simulink model "ACC_speed_change_curve_cs"  (R2016a)
settings: Solver=ode5  SolverMode=SingleTasking  StartTime=0.0  StopTime=inf  FixedStep=1/1000  RelTol=1e-3
PreLoadFcn:
  | mbxruntime.callbacks.PreLoadFcn(bdroot);
  | check_NUTS_defined;
  | 
  | assignin('base',['model_closed_' bdroot],false);addpath('../includes_ACC');
PostLoadFcn:
  | mbxruntime.callbacks.PostLoadFcn(bdroot);
InitFcn:
  | mbxruntime.callbacks.InitFcn(bdroot);
StartFcn:
  | mbxruntime.callbacks.StartFcn(bdroot);
StopFcn:
  | mbxruntime.callbacks.StopFcn(bdroot);
model workspace (MAT data in the model file):
  mbox_table : struct (value not decoded)
  model_closed = 0
  sim_status = 0
undefined symbols (not defined in the file or in its folder): DiscIntNeverNeededParam
undefined symbols (not defined in the file): SteeringColumn, SteeringWheel, WheelL0, WheelL1, WheelR0, WheelR1
libraries: simulink_extras x49, simulink x29, PreScanSimulinkLibrary x24, PreScanUsefulBlocks x2, Solver_SF x1, simulink_need_slupdate x1
(part 9 of 17)

== system ACC_speed_change_curve_cs/Toyota_Yaris_1/SteeringColumn_pivot_Mux ==
  X [m] : Inport
  Y [m] : Inport  Port=2
  Z [m] : Inport  Port=3
  Roll [rad] : Inport  Port=4
  Pitch [rad] : Inport  Port=5
  Yaw [rad] : Inport  Port=6
  Bus Creator : BusCreator  Inputs=3  OutDataTypeStr=Bus: PRESCAN_XYZ_DATA
  Bus Creator1 : BusCreator  Inputs=3  OutDataTypeStr=Bus: PRESCAN_RPY_DATA
  Bus Creator2 : BusCreator  Inputs=2  OutDataTypeStr=Bus: PRESCAN_POSE_DATA
  Joint : Outport
  wires:
  Yaw [rad]/1 -> Bus Creator1/3  "Yaw"
  Bus Creator1/1 -> Bus Creator2/2  "ORIENTATION"
  Bus Creator/1 -> Bus Creator2/1  "POSITION"
  X [m]/1 -> Bus Creator/1  "X"
  Y [m]/1 -> Bus Creator/2  "Y"
  Z [m]/1 -> Bus Creator/3  "Z"
  Bus Creator2/1 -> Joint/1
  Roll [rad]/1 -> Bus Creator1/1  "Roll"
  Pitch [rad]/1 -> Bus Creator1/2  "Pitch"

== system ACC_speed_change_curve_cs/Toyota_Yaris_1/SteeringWheel_pivot_Mux ==
  X [m] : Inport
  Y [m] : Inport  Port=2
  Z [m] : Inport  Port=3
  Roll [rad] : Inport  Port=4
  Pitch [rad] : Inport  Port=5
  Yaw [rad] : Inport  Port=6
  Bus Creator : BusCreator  Inputs=3  OutDataTypeStr=Bus: PRESCAN_XYZ_DATA
  Bus Creator1 : BusCreator  Inputs=3  OutDataTypeStr=Bus: PRESCAN_RPY_DATA
  Bus Creator2 : BusCreator  Inputs=2  OutDataTypeStr=Bus: PRESCAN_POSE_DATA
  Joint : Outport
  wires:
  Yaw [rad]/1 -> Bus Creator1/3  "Yaw"
  Bus Creator1/1 -> Bus Creator2/2  "ORIENTATION"
  Bus Creator/1 -> Bus Creator2/1  "POSITION"
  X [m]/1 -> Bus Creator/1  "X"
  Y [m]/1 -> Bus Creator/2  "Y"
  Z [m]/1 -> Bus Creator/3  "Z"
  Bus Creator2/1 -> Joint/1
  Roll [rad]/1 -> Bus Creator1/1  "Roll"
  Pitch [rad]/1 -> Bus Creator1/2  "Pitch"

== system ACC_speed_change_curve_cs/Toyota_Yaris_1/Trajectories ==
  Traj2State1 : Subsystem  Tag=Traj2State  mask(PreScan Demux Block:){}
      settings: DeleteFcn=PreScanBlockDeleteFcn;
  TrajCoGOffset : Subsystem  Tag=TrajCoGOffset  mask(Trajectory CoG Offset block){CoGOffsetZ=0.57, InitRoll=0, InitPitch=0}
      mask prompts: CoGOffsetZ "Z-component of CoG Offset [m]:"; InitRoll "Initial Roll angle [deg]:"; InitPitch "Initial Pitch angle [deg]:"
      mask help: A trajectory follows the surface of the road. However the position of a actor is based on the actor's Center of Gravity, which is typically above the road. This block converts from the trajectory along the road surface to the trajectory of the actor's CoG by realigning the z-component of the CoG offset to be normal to the road.
      settings: DeleteFcn=PreScanBlockDeleteFcn;
  Trajectory_4 : Subsystem  Tag=Trajectory  mask(PreScan Source Block: Trajectory){FileName='Trajectory_4.mat', TimeStep=20/1000}
      mask prompts: TimeStep "Time Step [s]"
      mask help:
      | The Trajectory block contains the trajectories defined in the PreScan Experiment Editor. The output of the trajectory block is the (vehicle) State.
      |
      | For more information, please click Help.
      mask init: same as ACC_speed_change_curve_cs/Audi_A8_1/Trajectories/Trajectory_1
      settings: DeleteFcn=PreScanBlockDeleteFcn;
      mask Help: eval('openHelp(312)')
      mask Display: fprintf(FileName)
  Trajectory_4_Offset : Constant  Tag=TrajectoryOffset  Value="[0  0  0  0  0  0]"
  State : Outport  Tag=TrajOutport
  wires:
  Trajectory_4/1(trajectory) -> Traj2State1/1(Traj Org)
  Trajectory_4_Offset/1 -> Traj2State1/2(Offset)
  TrajCoGOffset/1(State Out) -> State/1
  Traj2State1/1(state) -> TrajCoGOffset/1(State In)

== system ACC_speed_change_curve_cs/Toyota_Yaris_1/WheelDisplacement_Mux ==
  Steering Angle Front [rad] : Inport  Tag=inport/JointGroup  SampleTime=20/1000  BusOutputAsStruct=on
  Steering Angle Rear [rad] : Inport  Tag=inport/JointGroup  Port=2  SampleTime=20/1000  BusOutputAsStruct=on
  Rotation [rad] : Inport  Tag=inport/JointGroup  Port=3  SampleTime=20/1000  BusOutputAsStruct=on
  zDisp FL [m] : Inport  Tag=inport/JointGroup  Port=4  SampleTime=20/1000  BusOutputAsStruct=on
  zDisp FR [m] : Inport  Tag=inport/JointGroup  Port=5  SampleTime=20/1000  BusOutputAsStruct=on
  zDisp RL [m] : Inport  Tag=inport/JointGroup  Port=6  SampleTime=20/1000  BusOutputAsStruct=on
  zDisp RR [m] : Inport  Tag=inport/JointGroup  Port=7  SampleTime=20/1000  BusOutputAsStruct=on
  Ground_{1..12} (12 alike) : Ground
  WheelL0_Mux : Subsystem  Tag=mux/Joint  mask(PreScan Mux Block){DisplayName=WheelL0}
      mask prompts: DisplayName "Display Name"
      mask help:
      | This block simulates a generic joint used for generic models. This joint can be enabled/disabled from the GUI.
      |
      | For more information, please click Help.
      settings: DeleteFcn=PreScanBlockDeleteFcn;
      mask Help: eval('openHelp(254)')
  WheelL1_Mux : Subsystem  Tag=mux/Joint  mask(PreScan Mux Block){DisplayName=WheelL1}
      mask prompts: DisplayName "Display Name"
      mask help:
      | This block simulates a generic joint used for generic models. This joint can be enabled/disabled from the GUI.
      |
      | For more information, please click Help.
      settings: DeleteFcn=PreScanBlockDeleteFcn;
      mask Help: eval('openHelp(254)')
  WheelR0_Mux : Subsystem  Tag=mux/Joint  mask(PreScan Mux Block){DisplayName=WheelR0}
      mask prompts: DisplayName "Display Name"
      mask help:
      | This block simulates a generic joint used for generic models. This joint can be enabled/disabled from the GUI.
      |
      | For more information, please click Help.
      settings: DeleteFcn=PreScanBlockDeleteFcn;
      mask Help: eval('openHelp(254)')
  WheelR1_Mux : Subsystem  Tag=mux/Joint  mask(PreScan Mux Block){DisplayName=WheelR1}
      mask prompts: DisplayName "Display Name"
      mask help:
      | This block simulates a generic joint used for generic models. This joint can be enabled/disabled from the GUI.
      |
      | For more information, please click Help.
      settings: DeleteFcn=PreScanBlockDeleteFcn;
      mask Help: eval('openHelp(254)')
  WheelL0_Toyota_Yaris_1 : Outport  Tag=outport/JointActuator  OutDataTypeStr=Bus: PRESCAN_POSE_DATA  SampleTime=20/1000
  WheelL1_Toyota_Yaris_1 : Outport  Tag=outport/JointActuator  Port=2  OutDataTypeStr=Bus: PRESCAN_POSE_DATA  SampleTime=20/1000
  WheelR0_Toyota_Yaris_1 : Outport  Tag=outport/JointActuator  Port=3  OutDataTypeStr=Bus: PRESCAN_POSE_DATA  SampleTime=20/1000
  WheelR1_Toyota_Yaris_1 : Outport  Tag=outport/JointActuator  Port=4  OutDataTypeStr=Bus: PRESCAN_POSE_DATA  SampleTime=20/1000
  wires:
  WheelL0_Mux/1(Joint) -> WheelL0_Toyota_Yaris_1/1
  WheelL1_Mux/1(Joint) -> WheelL1_Toyota_Yaris_1/1
  WheelR0_Mux/1(Joint) -> WheelR0_Toyota_Yaris_1/1
  WheelR1_Mux/1(Joint) -> WheelR1_Toyota_Yaris_1/1
  Steering Angle Front [rad]/1 -> WheelR0_Mux/6(Yaw [rad]), WheelL0_Mux/6(Yaw [rad])
  Steering Angle Rear [rad]/1 -> WheelR1_Mux/6(Yaw [rad]), WheelL1_Mux/6(Yaw [rad])
  Rotation [rad]/1 -> WheelR0_Mux/5(Pitch [rad]), WheelL0_Mux/5(Pitch [rad]), WheelR1_Mux/5(Pitch [rad]), WheelL1_Mux/5(Pitch [rad])
  zDisp FL [m]/1 -> WheelL0_Mux/3(Z [m])
  zDisp FR [m]/1 -> WheelR0_Mux/3(Z [m])
  zDisp RL [m]/1 -> WheelL1_Mux/3(Z [m])
  zDisp RR [m]/1 -> WheelR1_Mux/3(Z [m])
  Ground_1/1 -> WheelL0_Mux/1(X [m])
  Ground_2/1 -> WheelL0_Mux/2(Y [m])
  Ground_3/1 -> WheelL0_Mux/4(Roll [rad])
  Ground_4/1 -> WheelL1_Mux/1(X [m])
  Ground_5/1 -> WheelL1_Mux/2(Y [m])
  Ground_6/1 -> WheelL1_Mux/4(Roll [rad])
  Ground_7/1 -> WheelR0_Mux/1(X [m])
  Ground_8/1 -> WheelR0_Mux/2(Y [m])
  Ground_9/1 -> WheelR0_Mux/4(Roll [rad])
  Ground_10/1 -> WheelR1_Mux/1(X [m])
  Ground_11/1 -> WheelR1_Mux/2(Y [m])
  Ground_12/1 -> WheelR1_Mux/4(Roll [rad])

== system ACC_speed_change_curve_cs/Toyota_Yaris_1/d2r SteeringColumn_pivot_Mux ==
  Degrees in : Inport
  Gain1 : Gain  Gain=pi/180  SaturateOnIntegerOverflow=on  OutDataTypeStr=Inherit: Same as input  ParamDataTypeStr=Inherit: Same as input
  Radians out : Outport  InitialOutput=0
  wires:
  Gain1/1 -> Radians out/1
  Degrees in/1 -> Gain1/1

== system ACC_speed_change_curve_cs/Toyota_Yaris_1/d2r SteeringWheel_pivot_Mux ==
  Degrees in : Inport
  Gain1 : Gain  Gain=pi/180  SaturateOnIntegerOverflow=on  OutDataTypeStr=Inherit: Same as input  ParamDataTypeStr=Inherit: Same as input
  Radians out : Outport  InitialOutput=0
  wires:
  Gain1/1 -> Radians out/1
  Degrees in/1 -> Gain1/1

== system ACC_speed_change_curve_cs/Toyota_Yaris_1/d2r WheelDisplacement_Mux 1 ==
  Degrees in : Inport
  Gain1 : Gain  Gain=pi/180  SaturateOnIntegerOverflow=on  OutDataTypeStr=Inherit: Same as input  ParamDataTypeStr=Inherit: Same as input
  Radians out : Outport  InitialOutput=0
  wires:
  Gain1/1 -> Radians out/1
  Degrees in/1 -> Gain1/1

== system ACC_speed_change_curve_cs/Toyota_Yaris_1/d2r WheelDisplacement_Mux 2 ==
  Degrees in : Inport
  Gain1 : Gain  Gain=pi/180  SaturateOnIntegerOverflow=on  OutDataTypeStr=Inherit: Same as input  ParamDataTypeStr=Inherit: Same as input
  Radians out : Outport  InitialOutput=0
  wires:
  Gain1/1 -> Radians out/1
  Degrees in/1 -> Gain1/1

== system ACC_speed_change_curve_cs/WheelL0_Audi_A8_1/Actuator ==
  Joint : Inport
  Bus Selector : BusSelector  OutputSignals=POSITION,ORIENTATION
  visu_Rotate : Subsystem  mask(RPYActuator){UniqueID=UniqueID, Object3DID=Rotate_ObjectID3D, TimeStep=TimeStep}
      mask prompts: UniqueID "Auto-Assigned: Unique ID"; Object3DID "Auto-Assigned: Child 3D Object ID"; TimeStep "Auto-Assigned: Upload Period [s]"
      mask help: Applies angles update to selected child object
      mask Help:
      | Applies position update to selected child object
      | 
      | - UniqueID (double)   : Unique ID of the parent actor
      | - Object3DID (string) : Name of the child 3D object
      mask Display: port_label('input', 1, ['visu_Rotate_' Object3DID])
  visu_Translate : Subsystem  mask(PositionActuator){UniqueID=UniqueID, Object3DID=Translate_ObjectID3D, TimeStep=TimeStep}
      mask prompts: UniqueID "Auto-Assigned: Unique ID"; Object3DID "Auto-Assigned: Child 3D Object ID"; TimeStep "Auto-Assigned: Upload Period [s]"
      mask help: Applies position update to selected child object
      mask Help:
      | Applies position update to selected child object
      | 
      | - UniqueID (double)   : Unique ID of the parent actor
      | - Object3DID (string) : Name of the child 3D object
      mask Display: port_label('input', 1, ['visu_Translate_' Object3DID])
  wires:
  Bus Selector/2 -> visu_Rotate/1(In1)  "<ORIENTATION>"
  Bus Selector/1 -> visu_Translate/1(In1)  "<POSITION>"
  Joint/1 -> Bus Selector/1

== system ACC_speed_change_curve_cs/WheelL0_BMW_X5_1/Actuator ==
  Joint : Inport
  Bus Selector : BusSelector  OutputSignals=POSITION,ORIENTATION
  visu_Rotate : Subsystem  mask(RPYActuator){UniqueID=UniqueID, Object3DID=Rotate_ObjectID3D, TimeStep=TimeStep}
      mask prompts: UniqueID "Auto-Assigned: Unique ID"; Object3DID "Auto-Assigned: Child 3D Object ID"; TimeStep "Auto-Assigned: Upload Period [s]"
      mask help: Applies angles update to selected child object
      mask Help:
      | Applies position update to selected child object
      | 
      | - UniqueID (double)   : Unique ID of the parent actor
      | - Object3DID (string) : Name of the child 3D object
      mask Display: port_label('input', 1, ['visu_Rotate_' Object3DID])
  visu_Translate : Subsystem  mask(PositionActuator){UniqueID=UniqueID, Object3DID=Translate_ObjectID3D, TimeStep=TimeStep}
      mask prompts: UniqueID "Auto-Assigned: Unique ID"; Object3DID "Auto-Assigned: Child 3D Object ID"; TimeStep "Auto-Assigned: Upload Period [s]"
      mask help: Applies position update to selected child object
      mask Help:
      | Applies position update to selected child object
      | 
      | - UniqueID (double)   : Unique ID of the parent actor
      | - Object3DID (string) : Name of the child 3D object
      mask Display: port_label('input', 1, ['visu_Translate_' Object3DID])
  wires:
  Bus Selector/2 -> visu_Rotate/1(In1)  "<ORIENTATION>"
  Bus Selector/1 -> visu_Translate/1(In1)  "<POSITION>"
  Joint/1 -> Bus Selector/1

== system ACC_speed_change_curve_cs/WheelL0_Toyota_Previa_1/Actuator ==
  Joint : Inport
  Bus Selector : BusSelector  OutputSignals=POSITION,ORIENTATION
  visu_Rotate : Subsystem  mask(RPYActuator){UniqueID=UniqueID, Object3DID=Rotate_ObjectID3D, TimeStep=TimeStep}
      mask prompts: UniqueID "Auto-Assigned: Unique ID"; Object3DID "Auto-Assigned: Child 3D Object ID"; TimeStep "Auto-Assigned: Upload Period [s]"
      mask help: Applies angles update to selected child object
      mask Help:
      | Applies position update to selected child object
      | 
      | - UniqueID (double)   : Unique ID of the parent actor
      | - Object3DID (string) : Name of the child 3D object
      mask Display: port_label('input', 1, ['visu_Rotate_' Object3DID])
  visu_Translate : Subsystem  mask(PositionActuator){UniqueID=UniqueID, Object3DID=Translate_ObjectID3D, TimeStep=TimeStep}
      mask prompts: UniqueID "Auto-Assigned: Unique ID"; Object3DID "Auto-Assigned: Child 3D Object ID"; TimeStep "Auto-Assigned: Upload Period [s]"
      mask help: Applies position update to selected child object
      mask Help:
      | Applies position update to selected child object
      | 
      | - UniqueID (double)   : Unique ID of the parent actor
      | - Object3DID (string) : Name of the child 3D object
      mask Display: port_label('input', 1, ['visu_Translate_' Object3DID])
  wires:
  Bus Selector/2 -> visu_Rotate/1(In1)  "<ORIENTATION>"
  Bus Selector/1 -> visu_Translate/1(In1)  "<POSITION>"
  Joint/1 -> Bus Selector/1

== system ACC_speed_change_curve_cs/WheelL0_Toyota_Yaris_1/Actuator ==
  Joint : Inport
  Bus Selector : BusSelector  OutputSignals=POSITION,ORIENTATION
  visu_Rotate : Subsystem  mask(RPYActuator){UniqueID=UniqueID, Object3DID=Rotate_ObjectID3D, TimeStep=TimeStep}
      mask prompts: UniqueID "Auto-Assigned: Unique ID"; Object3DID "Auto-Assigned: Child 3D Object ID"; TimeStep "Auto-Assigned: Upload Period [s]"
      mask help: Applies angles update to selected child object
      mask Help:
      | Applies position update to selected child object
      | 
      | - UniqueID (double)   : Unique ID of the parent actor
      | - Object3DID (string) : Name of the child 3D object
      mask Display: port_label('input', 1, ['visu_Rotate_' Object3DID])
  visu_Translate : Subsystem  mask(PositionActuator){UniqueID=UniqueID, Object3DID=Translate_ObjectID3D, TimeStep=TimeStep}
      mask prompts: UniqueID "Auto-Assigned: Unique ID"; Object3DID "Auto-Assigned: Child 3D Object ID"; TimeStep "Auto-Assigned: Upload Period [s]"
      mask help: Applies position update to selected child object
      mask Help:
      | Applies position update to selected child object
      | 
      | - UniqueID (double)   : Unique ID of the parent actor
      | - Object3DID (string) : Name of the child 3D object
      mask Display: port_label('input', 1, ['visu_Translate_' Object3DID])
  wires:
  Bus Selector/2 -> visu_Rotate/1(In1)  "<ORIENTATION>"
  Bus Selector/1 -> visu_Translate/1(In1)  "<POSITION>"
  Joint/1 -> Bus Selector/1

== system ACC_speed_change_curve_cs/WheelL1_Audi_A8_1/Actuator ==
  Joint : Inport
  Bus Selector : BusSelector  OutputSignals=POSITION,ORIENTATION
  visu_Rotate : Subsystem  mask(RPYActuator){UniqueID=UniqueID, Object3DID=Rotate_ObjectID3D, TimeStep=TimeStep}
      mask prompts: UniqueID "Auto-Assigned: Unique ID"; Object3DID "Auto-Assigned: Child 3D Object ID"; TimeStep "Auto-Assigned: Upload Period [s]"
      mask help: Applies angles update to selected child object
      mask Help:
      | Applies position update to selected child object
      | 
      | - UniqueID (double)   : Unique ID of the parent actor
      | - Object3DID (string) : Name of the child 3D object
      mask Display: port_label('input', 1, ['visu_Rotate_' Object3DID])
  visu_Translate : Subsystem  mask(PositionActuator){UniqueID=UniqueID, Object3DID=Translate_ObjectID3D, TimeStep=TimeStep}
      mask prompts: UniqueID "Auto-Assigned: Unique ID"; Object3DID "Auto-Assigned: Child 3D Object ID"; TimeStep "Auto-Assigned: Upload Period [s]"
      mask help: Applies position update to selected child object
      mask Help:
      | Applies position update to selected child object
      | 
      | - UniqueID (double)   : Unique ID of the parent actor
      | - Object3DID (string) : Name of the child 3D object
      mask Display: port_label('input', 1, ['visu_Translate_' Object3DID])
  wires:
  Bus Selector/2 -> visu_Rotate/1(In1)  "<ORIENTATION>"
  Bus Selector/1 -> visu_Translate/1(In1)  "<POSITION>"
  Joint/1 -> Bus Selector/1

== system ACC_speed_change_curve_cs/WheelL1_BMW_X5_1/Actuator ==
  Joint : Inport
  Bus Selector : BusSelector  OutputSignals=POSITION,ORIENTATION
  visu_Rotate : Subsystem  mask(RPYActuator){UniqueID=UniqueID, Object3DID=Rotate_ObjectID3D, TimeStep=TimeStep}
      mask prompts: UniqueID "Auto-Assigned: Unique ID"; Object3DID "Auto-Assigned: Child 3D Object ID"; TimeStep "Auto-Assigned: Upload Period [s]"
      mask help: Applies angles update to selected child object
      mask Help:
      | Applies position update to selected child object
      | 
      | - UniqueID (double)   : Unique ID of the parent actor
      | - Object3DID (string) : Name of the child 3D object
      mask Display: port_label('input', 1, ['visu_Rotate_' Object3DID])
  visu_Translate : Subsystem  mask(PositionActuator){UniqueID=UniqueID, Object3DID=Translate_ObjectID3D, TimeStep=TimeStep}
      mask prompts: UniqueID "Auto-Assigned: Unique ID"; Object3DID "Auto-Assigned: Child 3D Object ID"; TimeStep "Auto-Assigned: Upload Period [s]"
      mask help: Applies position update to selected child object
      mask Help:
      | Applies position update to selected child object
      | 
      | - UniqueID (double)   : Unique ID of the parent actor
      | - Object3DID (string) : Name of the child 3D object
      mask Display: port_label('input', 1, ['visu_Translate_' Object3DID])
  wires:
  Bus Selector/2 -> visu_Rotate/1(In1)  "<ORIENTATION>"
  Bus Selector/1 -> visu_Translate/1(In1)  "<POSITION>"
  Joint/1 -> Bus Selector/1

== system ACC_speed_change_curve_cs/WheelL1_Toyota_Previa_1/Actuator ==
  Joint : Inport
  Bus Selector : BusSelector  OutputSignals=POSITION,ORIENTATION
  visu_Rotate : Subsystem  mask(RPYActuator){UniqueID=UniqueID, Object3DID=Rotate_ObjectID3D, TimeStep=TimeStep}
      mask prompts: UniqueID "Auto-Assigned: Unique ID"; Object3DID "Auto-Assigned: Child 3D Object ID"; TimeStep "Auto-Assigned: Upload Period [s]"
      mask help: Applies angles update to selected child object
      mask Help:
      | Applies position update to selected child object
      | 
      | - UniqueID (double)   : Unique ID of the parent actor
      | - Object3DID (string) : Name of the child 3D object
      mask Display: port_label('input', 1, ['visu_Rotate_' Object3DID])
  visu_Translate : Subsystem  mask(PositionActuator){UniqueID=UniqueID, Object3DID=Translate_ObjectID3D, TimeStep=TimeStep}
      mask prompts: UniqueID "Auto-Assigned: Unique ID"; Object3DID "Auto-Assigned: Child 3D Object ID"; TimeStep "Auto-Assigned: Upload Period [s]"
      mask help: Applies position update to selected child object
      mask Help:
      | Applies position update to selected child object
      | 
      | - UniqueID (double)   : Unique ID of the parent actor
      | - Object3DID (string) : Name of the child 3D object
      mask Display: port_label('input', 1, ['visu_Translate_' Object3DID])
  wires:
  Bus Selector/2 -> visu_Rotate/1(In1)  "<ORIENTATION>"
  Bus Selector/1 -> visu_Translate/1(In1)  "<POSITION>"
  Joint/1 -> Bus Selector/1

== system ACC_speed_change_curve_cs/WheelL1_Toyota_Yaris_1/Actuator ==
  Joint : Inport
  Bus Selector : BusSelector  OutputSignals=POSITION,ORIENTATION
  visu_Rotate : Subsystem  mask(RPYActuator){UniqueID=UniqueID, Object3DID=Rotate_ObjectID3D, TimeStep=TimeStep}
      mask prompts: UniqueID "Auto-Assigned: Unique ID"; Object3DID "Auto-Assigned: Child 3D Object ID"; TimeStep "Auto-Assigned: Upload Period [s]"
      mask help: Applies angles update to selected child object
      mask Help:
      | Applies position update to selected child object
      | 
      | - UniqueID (double)   : Unique ID of the parent actor
      | - Object3DID (string) : Name of the child 3D object
      mask Display: port_label('input', 1, ['visu_Rotate_' Object3DID])
  visu_Translate : Subsystem  mask(PositionActuator){UniqueID=UniqueID, Object3DID=Translate_ObjectID3D, TimeStep=TimeStep}
      mask prompts: UniqueID "Auto-Assigned: Unique ID"; Object3DID "Auto-Assigned: Child 3D Object ID"; TimeStep "Auto-Assigned: Upload Period [s]"
      mask help: Applies position update to selected child object
      mask Help:
      | Applies position update to selected child object
      | 
      | - UniqueID (double)   : Unique ID of the parent actor
      | - Object3DID (string) : Name of the child 3D object
      mask Display: port_label('input', 1, ['visu_Translate_' Object3DID])
  wires:
  Bus Selector/2 -> visu_Rotate/1(In1)  "<ORIENTATION>"
  Bus Selector/1 -> visu_Translate/1(In1)  "<POSITION>"
  Joint/1 -> Bus Selector/1

== system ACC_speed_change_curve_cs/WheelR0_Audi_A8_1/Actuator ==
  Joint : Inport
  Bus Selector : BusSelector  OutputSignals=POSITION,ORIENTATION
  visu_Rotate : Subsystem  mask(RPYActuator){UniqueID=UniqueID, Object3DID=Rotate_ObjectID3D, TimeStep=TimeStep}
      mask prompts: UniqueID "Auto-Assigned: Unique ID"; Object3DID "Auto-Assigned: Child 3D Object ID"; TimeStep "Auto-Assigned: Upload Period [s]"
      mask help: Applies angles update to selected child object
      mask Help:
      | Applies position update to selected child object
      | 
      | - UniqueID (double)   : Unique ID of the parent actor
      | - Object3DID (string) : Name of the child 3D object
      mask Display: port_label('input', 1, ['visu_Rotate_' Object3DID])
  visu_Translate : Subsystem  mask(PositionActuator){UniqueID=UniqueID, Object3DID=Translate_ObjectID3D, TimeStep=TimeStep}
      mask prompts: UniqueID "Auto-Assigned: Unique ID"; Object3DID "Auto-Assigned: Child 3D Object ID"; TimeStep "Auto-Assigned: Upload Period [s]"
      mask help: Applies position update to selected child object
      mask Help:
      | Applies position update to selected child object
      | 
      | - UniqueID (double)   : Unique ID of the parent actor
      | - Object3DID (string) : Name of the child 3D object
      mask Display: port_label('input', 1, ['visu_Translate_' Object3DID])
  wires:
  Bus Selector/2 -> visu_Rotate/1(In1)  "<ORIENTATION>"
  Bus Selector/1 -> visu_Translate/1(In1)  "<POSITION>"
  Joint/1 -> Bus Selector/1

== system ACC_speed_change_curve_cs/WheelR0_BMW_X5_1/Actuator ==
  Joint : Inport
  Bus Selector : BusSelector  OutputSignals=POSITION,ORIENTATION
  visu_Rotate : Subsystem  mask(RPYActuator){UniqueID=UniqueID, Object3DID=Rotate_ObjectID3D, TimeStep=TimeStep}
      mask prompts: UniqueID "Auto-Assigned: Unique ID"; Object3DID "Auto-Assigned: Child 3D Object ID"; TimeStep "Auto-Assigned: Upload Period [s]"
      mask help: Applies angles update to selected child object
      mask Help:
      | Applies position update to selected child object
      | 
      | - UniqueID (double)   : Unique ID of the parent actor
      | - Object3DID (string) : Name of the child 3D object
      mask Display: port_label('input', 1, ['visu_Rotate_' Object3DID])
  visu_Translate : Subsystem  mask(PositionActuator){UniqueID=UniqueID, Object3DID=Translate_ObjectID3D, TimeStep=TimeStep}
      mask prompts: UniqueID "Auto-Assigned: Unique ID"; Object3DID "Auto-Assigned: Child 3D Object ID"; TimeStep "Auto-Assigned: Upload Period [s]"
      mask help: Applies position update to selected child object
      mask Help:
      | Applies position update to selected child object
      | 
      | - UniqueID (double)   : Unique ID of the parent actor
      | - Object3DID (string) : Name of the child 3D object
      mask Display: port_label('input', 1, ['visu_Translate_' Object3DID])
  wires:
  Bus Selector/2 -> visu_Rotate/1(In1)  "<ORIENTATION>"
  Bus Selector/1 -> visu_Translate/1(In1)  "<POSITION>"
  Joint/1 -> Bus Selector/1

== system ACC_speed_change_curve_cs/WheelR0_Toyota_Previa_1/Actuator ==
  Joint : Inport
  Bus Selector : BusSelector  OutputSignals=POSITION,ORIENTATION
  visu_Rotate : Subsystem  mask(RPYActuator){UniqueID=UniqueID, Object3DID=Rotate_ObjectID3D, TimeStep=TimeStep}
      mask prompts: UniqueID "Auto-Assigned: Unique ID"; Object3DID "Auto-Assigned: Child 3D Object ID"; TimeStep "Auto-Assigned: Upload Period [s]"
      mask help: Applies angles update to selected child object
      mask Help:
      | Applies position update to selected child object
      | 
      | - UniqueID (double)   : Unique ID of the parent actor
      | - Object3DID (string) : Name of the child 3D object
      mask Display: port_label('input', 1, ['visu_Rotate_' Object3DID])
  visu_Translate : Subsystem  mask(PositionActuator){UniqueID=UniqueID, Object3DID=Translate_ObjectID3D, TimeStep=TimeStep}
      mask prompts: UniqueID "Auto-Assigned: Unique ID"; Object3DID "Auto-Assigned: Child 3D Object ID"; TimeStep "Auto-Assigned: Upload Period [s]"
      mask help: Applies position update to selected child object
      mask Help:
      | Applies position update to selected child object
      | 
      | - UniqueID (double)   : Unique ID of the parent actor
      | - Object3DID (string) : Name of the child 3D object
      mask Display: port_label('input', 1, ['visu_Translate_' Object3DID])
  wires:
  Bus Selector/2 -> visu_Rotate/1(In1)  "<ORIENTATION>"
  Bus Selector/1 -> visu_Translate/1(In1)  "<POSITION>"
  Joint/1 -> Bus Selector/1

== system ACC_speed_change_curve_cs/WheelR0_Toyota_Yaris_1/Actuator ==
  Joint : Inport
  Bus Selector : BusSelector  OutputSignals=POSITION,ORIENTATION
  visu_Rotate : Subsystem  mask(RPYActuator){UniqueID=UniqueID, Object3DID=Rotate_ObjectID3D, TimeStep=TimeStep}
      mask prompts: UniqueID "Auto-Assigned: Unique ID"; Object3DID "Auto-Assigned: Child 3D Object ID"; TimeStep "Auto-Assigned: Upload Period [s]"
      mask help: Applies angles update to selected child object
      mask Help:
      | Applies position update to selected child object
      | 
      | - UniqueID (double)   : Unique ID of the parent actor
      | - Object3DID (string) : Name of the child 3D object
      mask Display: port_label('input', 1, ['visu_Rotate_' Object3DID])
  visu_Translate : Subsystem  mask(PositionActuator){UniqueID=UniqueID, Object3DID=Translate_ObjectID3D, TimeStep=TimeStep}
      mask prompts: UniqueID "Auto-Assigned: Unique ID"; Object3DID "Auto-Assigned: Child 3D Object ID"; TimeStep "Auto-Assigned: Upload Period [s]"
      mask help: Applies position update to selected child object
      mask Help:
      | Applies position update to selected child object
      | 
      | - UniqueID (double)   : Unique ID of the parent actor
      | - Object3DID (string) : Name of the child 3D object
      mask Display: port_label('input', 1, ['visu_Translate_' Object3DID])
  wires:
  Bus Selector/2 -> visu_Rotate/1(In1)  "<ORIENTATION>"
  Bus Selector/1 -> visu_Translate/1(In1)  "<POSITION>"
  Joint/1 -> Bus Selector/1

== system ACC_speed_change_curve_cs/WheelR1_Audi_A8_1/Actuator ==
  Joint : Inport
  Bus Selector : BusSelector  OutputSignals=POSITION,ORIENTATION
  visu_Rotate : Subsystem  mask(RPYActuator){UniqueID=UniqueID, Object3DID=Rotate_ObjectID3D, TimeStep=TimeStep}
      mask prompts: UniqueID "Auto-Assigned: Unique ID"; Object3DID "Auto-Assigned: Child 3D Object ID"; TimeStep "Auto-Assigned: Upload Period [s]"
      mask help: Applies angles update to selected child object
      mask Help:
      | Applies position update to selected child object
      | 
      | - UniqueID (double)   : Unique ID of the parent actor
      | - Object3DID (string) : Name of the child 3D object
      mask Display: port_label('input', 1, ['visu_Rotate_' Object3DID])
  visu_Translate : Subsystem  mask(PositionActuator){UniqueID=UniqueID, Object3DID=Translate_ObjectID3D, TimeStep=TimeStep}
      mask prompts: UniqueID "Auto-Assigned: Unique ID"; Object3DID "Auto-Assigned: Child 3D Object ID"; TimeStep "Auto-Assigned: Upload Period [s]"
      mask help: Applies position update to selected child object
      mask Help:
      | Applies position update to selected child object
      | 
      | - UniqueID (double)   : Unique ID of the parent actor
      | - Object3DID (string) : Name of the child 3D object
      mask Display: port_label('input', 1, ['visu_Translate_' Object3DID])
  wires:
  Bus Selector/2 -> visu_Rotate/1(In1)  "<ORIENTATION>"
  Bus Selector/1 -> visu_Translate/1(In1)  "<POSITION>"
  Joint/1 -> Bus Selector/1

== system ACC_speed_change_curve_cs/WheelR1_BMW_X5_1/Actuator ==
  Joint : Inport
  Bus Selector : BusSelector  OutputSignals=POSITION,ORIENTATION
  visu_Rotate : Subsystem  mask(RPYActuator){UniqueID=UniqueID, Object3DID=Rotate_ObjectID3D, TimeStep=TimeStep}
      mask prompts: UniqueID "Auto-Assigned: Unique ID"; Object3DID "Auto-Assigned: Child 3D Object ID"; TimeStep "Auto-Assigned: Upload Period [s]"
      mask help: Applies angles update to selected child object
      mask Help:
      | Applies position update to selected child object
      | 
      | - UniqueID (double)   : Unique ID of the parent actor
      | - Object3DID (string) : Name of the child 3D object
      mask Display: port_label('input', 1, ['visu_Rotate_' Object3DID])
  visu_Translate : Subsystem  mask(PositionActuator){UniqueID=UniqueID, Object3DID=Translate_ObjectID3D, TimeStep=TimeStep}
      mask prompts: UniqueID "Auto-Assigned: Unique ID"; Object3DID "Auto-Assigned: Child 3D Object ID"; TimeStep "Auto-Assigned: Upload Period [s]"
      mask help: Applies position update to selected child object
      mask Help:
      | Applies position update to selected child object
      | 
      | - UniqueID (double)   : Unique ID of the parent actor
      | - Object3DID (string) : Name of the child 3D object
      mask Display: port_label('input', 1, ['visu_Translate_' Object3DID])
  wires:
  Bus Selector/2 -> visu_Rotate/1(In1)  "<ORIENTATION>"
  Bus Selector/1 -> visu_Translate/1(In1)  "<POSITION>"
  Joint/1 -> Bus Selector/1

== system ACC_speed_change_curve_cs/WheelR1_Toyota_Previa_1/Actuator ==
  Joint : Inport
  Bus Selector : BusSelector  OutputSignals=POSITION,ORIENTATION
  visu_Rotate : Subsystem  mask(RPYActuator){UniqueID=UniqueID, Object3DID=Rotate_ObjectID3D, TimeStep=TimeStep}
      mask prompts: UniqueID "Auto-Assigned: Unique ID"; Object3DID "Auto-Assigned: Child 3D Object ID"; TimeStep "Auto-Assigned: Upload Period [s]"
      mask help: Applies angles update to selected child object
      mask Help:
      | Applies position update to selected child object
      | 
      | - UniqueID (double)   : Unique ID of the parent actor
      | - Object3DID (string) : Name of the child 3D object
      mask Display: port_label('input', 1, ['visu_Rotate_' Object3DID])
  visu_Translate : Subsystem  mask(PositionActuator){UniqueID=UniqueID, Object3DID=Translate_ObjectID3D, TimeStep=TimeStep}
      mask prompts: UniqueID "Auto-Assigned: Unique ID"; Object3DID "Auto-Assigned: Child 3D Object ID"; TimeStep "Auto-Assigned: Upload Period [s]"
      mask help: Applies position update to selected child object
      mask Help:
      | Applies position update to selected child object
      | 
      | - UniqueID (double)   : Unique ID of the parent actor
      | - Object3DID (string) : Name of the child 3D object
      mask Display: port_label('input', 1, ['visu_Translate_' Object3DID])
  wires:
  Bus Selector/2 -> visu_Rotate/1(In1)  "<ORIENTATION>"
  Bus Selector/1 -> visu_Translate/1(In1)  "<POSITION>"
  Joint/1 -> Bus Selector/1

== system ACC_speed_change_curve_cs/WheelR1_Toyota_Yaris_1/Actuator ==
  Joint : Inport
  Bus Selector : BusSelector  OutputSignals=POSITION,ORIENTATION
  visu_Rotate : Subsystem  mask(RPYActuator){UniqueID=UniqueID, Object3DID=Rotate_ObjectID3D, TimeStep=TimeStep}
      mask prompts: UniqueID "Auto-Assigned: Unique ID"; Object3DID "Auto-Assigned: Child 3D Object ID"; TimeStep "Auto-Assigned: Upload Period [s]"
      mask help: Applies angles update to selected child object
      mask Help:
      | Applies position update to selected child object
      | 
      | - UniqueID (double)   : Unique ID of the parent actor
      | - Object3DID (string) : Name of the child 3D object
      mask Display: port_label('input', 1, ['visu_Rotate_' Object3DID])
  visu_Translate : Subsystem  mask(PositionActuator){UniqueID=UniqueID, Object3DID=Translate_ObjectID3D, TimeStep=TimeStep}
      mask prompts: UniqueID "Auto-Assigned: Unique ID"; Object3DID "Auto-Assigned: Child 3D Object ID"; TimeStep "Auto-Assigned: Upload Period [s]"
      mask help: Applies position update to selected child object
      mask Help:
      | Applies position update to selected child object
      | 
      | - UniqueID (double)   : Unique ID of the parent actor
      | - Object3DID (string) : Name of the child 3D object
      mask Display: port_label('input', 1, ['visu_Translate_' Object3DID])
  wires:
  Bus Selector/2 -> visu_Rotate/1(In1)  "<ORIENTATION>"
  Bus Selector/1 -> visu_Translate/1(In1)  "<POSITION>"
  Joint/1 -> Bus Selector/1

== system ACC_speed_change_curve_cs/Audi_A8_1/ACC_System/Rate transition from other signals ==
  In1 : Inport
  In2 : Inport  Port=2
  Rate Transition1 : RateTransition  Integrity=off  OutPortSampleTime=Tsensor
  Rate Transition2 : RateTransition  Integrity=off  OutPortSampleTime=Tsensor
  Out1 : Outport
  Out2 : Outport  Port=2
  wires:
  Rate Transition2/1 -> Out2/1
  In2/1 -> Rate Transition2/1
  Rate Transition1/1 -> Out1/1
  In1/1 -> Rate Transition1/1

== system ACC_speed_change_curve_cs/Audi_A8_1/ACC_System/Rate transition from EGO ==
  In1 : Inport
  In2 : Inport  Port=2
  Rate Transition1 : RateTransition  Integrity=off  OutPortSampleTime=Tsensor
  Rate Transition2 : RateTransition  Integrity=off  OutPortSampleTime=Tsensor
  Out1 : Outport
  Out2 : Outport  Port=2
  wires:
  In1/1 -> Rate Transition1/1
  Rate Transition1/1 -> Out1/1
  In2/1 -> Rate Transition2/1
  Rate Transition2/1 -> Out2/1

== system ACC_speed_change_curve_cs/Audi_A8_1/ACC_System/Rate transition from TIS1 ==
  In1 : Inport
  In2 : Inport  Port=2
  In3 : Inport  Port=3
  Rate Transition1 : RateTransition  Integrity=off  OutPortSampleTime=Tsensor
  Rate Transition2 : RateTransition  Integrity=off  OutPortSampleTime=Tsensor
  Rate Transition3 : RateTransition  Integrity=off  OutPortSampleTime=Tsensor
  Out1 : Outport
  Out2 : Outport  Port=2
  Out3 : Outport  Port=3
  wires:
  Rate Transition3/1 -> Out3/1
  In3/1 -> Rate Transition3/1
  Rate Transition2/1 -> Out2/1
  In2/1 -> Rate Transition2/1
  Rate Transition1/1 -> Out1/1
  In1/1 -> Rate Transition1/1

== system ACC_speed_change_curve_cs/Audi_A8_1/ACC_System/Rate transition from TIS2 ==
  In1 : Inport
  In2 : Inport  Port=2
  In3 : Inport  Port=3
  Rate Transition1 : RateTransition  Integrity=off  OutPortSampleTime=Tsensor
  Rate Transition2 : RateTransition  Integrity=off  OutPortSampleTime=Tsensor
  Rate Transition3 : RateTransition  Integrity=off  OutPortSampleTime=Tsensor
  Out1 : Outport
  Out2 : Outport  Port=2
  Out3 : Outport  Port=3
  wires:
  In1/1 -> Rate Transition3/1
  Rate Transition3/1 -> Out1/1
  In2/1 -> Rate Transition1/1
  Rate Transition1/1 -> Out2/1
  In3/1 -> Rate Transition2/1
  Rate Transition2/1 -> Out3/1

== system ACC_speed_change_curve_cs/Audi_A8_1/ACC_System/Switching TIS ==
  note: === Switching block ===
      |
      |  - determines if the EGO car is moving on a straight road or on a bend raod,
      |  - based on the actual value of the yaw rate of the EGO car.
  straight_mux : Inport
  EGO_Yaw_rate_[deg/s] : Inport  Port=2
  bend_mux : Inport  Port=3
  1deg_per_s : Constant
  Abs : Abs
  Relational Operator : RelationalOperator  Operator=<  OutDataTypeStr=boolean
  Selector : Selector  InputPortWidth=12  IndexOptions=Index vector (dialog)  Indices=[6 12]  OutputSizes=1
  Switch : Switch  Criteria=u2 ~= 0  Threshold=0.5
  demux : Outport
  indexes : Outport  Port=2
  wires:
  EGO_Yaw_rate_[deg/s]/1 -> Abs/1
  1deg_per_s/1 -> Relational Operator/2
  Relational Operator/1 -> Switch/2
  straight_mux/1 -> Switch/1
  Switch/1 -> demux/1, Selector/1
  bend_mux/1 -> Switch/3
  Abs/1 -> Relational Operator/1
  Selector/1 -> indexes/1

== system ACC_speed_change_curve_cs/Audi_A8_1/ACC_System/TIS1 Bend Road ==
  note: === TIS1 Bend Road block ===
      |
      |  - interpretes information provided from the first TIS sensor,
      |  - computes HeadWay Time (HWT) for object on the lane of the EGO car on the bend road,
      |  - determines if detected objects is potentially dengerous,
      |  - outputs distance to the following car, computes its velocity and safe distance to be kept.
  EGO_velocity [m/s] : Inport
  TIS1_range [m] : Inport  Port=2  PortDimensions=TISdet(1)
  TIS1_rangedot [m/s] : Inport  Port=3  PortDimensions=TISdet(1)
  TIS1_theta [deg] : Inport  Port=4  PortDimensions=TISdet(1)
  HWT_dem [s] : Inport  Port=5
  Standstill [m] : Inport  Port=6
  EGO_Yaw_rate [deg/s] : Inport  Port=7
  EGO_velocity [m/s]2 : InportShadow
  Embedded MATLAB Function : MATLAB Function  TreatAsAtomicUnit=on
  Hold : Subsystem
  Lead Car Longitudinal Velocity : Subsystem
  TIS1 Closest Object On Bend Road : Subsystem
  TIS1 HWT Computing : Subsystem
  TIS1 HWT Flag : Subsystem
  TIS1 Objects On Bend Road : Subsystem
  TIS1 Sorting  Fun : Subsystem
  HWT_flag : Outport
  TIS1 Lead distance [m] : Outport  Port=2
  TIS1 Safe_distance [m] : Outport  Port=3
  TIS1_HWT_bend : Outport  Port=4
  TIS1 lead velocity [m/s] : Outport  Port=5
  index : Outport  Port=6
  wires:
  TIS1_theta [deg]/1 -> TIS1 Sorting  Fun/3(TIS1theta [deg])
  TIS1_rangedot [m/s]/1 -> TIS1 Sorting  Fun/2(TIS1rangedot [m/s])
  TIS1_range [m]/1 -> TIS1 Sorting  Fun/1(TIS1range [m])
  TIS1 Sorting  Fun/1(TIS1_RANGE [m]) -> TIS1 Objects On Bend Road/1(TIS1_range [m])
  TIS1 Sorting  Fun/2(TIS1_RANGEDOT [m/s]) -> TIS1 Objects On Bend Road/2(TIS1_rangedot [m/s])
  TIS1 Sorting  Fun/3(TIS1_THETA [rad]) -> TIS1 Objects On Bend Road/3(TIS1_theta [rad])
  EGO_velocity [m/s]/1 -> TIS1 Objects On Bend Road/4(EGO_Velocity [m/s])
  EGO_Yaw_rate [deg/s]/1 -> TIS1 Objects On Bend Road/5(EGO_Yaw_rate_[deg/s])
  Embedded MATLAB Function/1(index) -> TIS1 Closest Object On Bend Road/1(index), index/1
  TIS1 Objects On Bend Road/1(TIS1_RANGE [m]) -> TIS1 Closest Object On Bend Road/2(TIS1_range [m]), Embedded MATLAB Function/1(distance)
  TIS1 Objects On Bend Road/2(TIS1_RANGEDOT [m/s]) -> TIS1 Closest Object On Bend Road/3(TIS1_rangedot [m])
  TIS1 Objects On Bend Road/3(TIS1_THETA [rad]) -> TIS1 Closest Object On Bend Road/4(TIS1_theta [rad])
  TIS1 Objects On Bend Road/4(TIS1_Distance [m]) -> TIS1 Closest Object On Bend Road/5(TIS1_Distance [m])
  TIS1 Objects On Bend Road/5(TIS1_lambda_[rad]) -> TIS1 Closest Object On Bend Road/6(TIS1_lambda [rad])
  TIS1 Closest Object On Bend Road/4(Distance [m]) -> TIS1 Lead distance [m]/1, TIS1 HWT Computing/1(Distance [m]), TIS1 HWT Flag/1(Distance closest [m])
  EGO_velocity [m/s]2/1 -> Lead Car Longitudinal Velocity/3(EGO Velocity [m/s]), TIS1 HWT Computing/2(Velocity [m/s])
  TIS1 Closest Object On Bend Road/2(rangedot [m/s]) -> Lead Car Longitudinal Velocity/2(TIS1 Rangedot [m/s])
  TIS1 HWT Computing/1(HWT [s]) -> TIS1_HWT_bend/1, TIS1 HWT Flag/2(HWT [s])
  HWT_dem [s]/1 -> Lead Car Longitudinal Velocity/1(HWT_dem (s)), TIS1 HWT Flag/3(HWT_dem [s])
  Standstill [m]/1 -> Lead Car Longitudinal Velocity/4(Standstill [m]), TIS1 HWT Flag/4(Standstill distance)
  TIS1 Closest Object On Bend Road/3(theta [rad]) -> Lead Car Longitudinal Velocity/5(theta [rad])
  TIS1 Closest Object On Bend Road/5(lambda [rad]) -> Lead Car Longitudinal Velocity/6(lambda [rad])
  Lead Car Longitudinal Velocity/1(Safe distance [m]) -> TIS1 Safe_distance [m]/1
  Lead Car Longitudinal Velocity/2(Lead velocity [m/s]) -> TIS1 lead velocity [m/s]/1, Hold/2(lead_vel_in)
  Hold/1(HWT_flag) -> HWT_flag/1
  TIS1 HWT Flag/1(HWT_flag) -> Hold/1(HWTflagIN)
  TIS1 Closest Object On Bend Road/1(range [m]) -> Lead Car Longitudinal Velocity/7(TIS1 Range [m])

== system ACC_speed_change_curve_cs/Audi_A8_1/ACC_System/TIS1 Straight Road ==
  note: === TIS1 Straight Road block ===
      |
      |  - interpretes information provided from the first TIS sensor,
      |  - computes HeadWay Time (HWT) for object on the lane in front of the EGO car,
      |  - determines if detected objects is potentially dengerous,
      |  - outputs distance to the following car, computes its velocity and safe distance to be kept.
  EGO_velocity [m/s] : Inport
  TIS1_range [m] : Inport  Port=2  PortDimensions=TISdet(1)
  TIS1_rangedot [m/s] : Inport  Port=3  PortDimensions=TISdet(1)
  TIS1_theta [deg] : Inport  Port=4  PortDimensions=TISdet(1)
  HWT_dem [s] : Inport  Port=5
  Standstill [m] : Inport  Port=6
  HWT_dem [s]1 : InportShadow  Port=5
  Hold : Subsystem
  TIS1 Closest Object : Subsystem
  TIS1 HWT Computing : Subsystem
  TIS1 HWT Computing1 : Subsystem
  TIS1 HWT Flag : Subsystem
  TIS1 Lead Car Longitudinal Velocity : Subsystem
  TIS1 Objects On Lane : Subsystem
  TIS1 Sorting Fun : Subsystem
  TIS1_closest_object_search : MATLAB Function  TreatAsAtomicUnit=on
  HWT_flag : Outport
  TIS1 Lead distance [m] : Outport  Port=2
  TIS1 Safe_distance [m] : Outport  Port=3
  TIS1_HWT_straight : Outport  Port=4
  TIS1 Lead velocity [m/s] : Outport  Port=5
  index : Outport  Port=6
  wires:
  TIS1_range [m]/1 -> TIS1 Sorting Fun/1(TIS1range [m])
  TIS1_rangedot [m/s]/1 -> TIS1 Sorting Fun/2(TIS1rangedot [m/s])
  TIS1_theta [deg]/1 -> TIS1 Sorting Fun/3(TIS1theta [deg])
  TIS1 Sorting Fun/1(TIS1_RANGE [m]) -> TIS1 Objects On Lane/1(TIS1_range [m])
  TIS1 Sorting Fun/2(TIS1_RANGEDOT [m/s]) -> TIS1 Objects On Lane/2(TIS1_rangedot [m/s])
  TIS1 Sorting Fun/3(TIS1_THETA [rad]) -> TIS1 Objects On Lane/3(TIS1_theta [rad])
  TIS1_closest_object_search/1(index) -> TIS1 Closest Object/3(index), index/1
  TIS1 HWT Computing/1(HWT [s]) -> TIS1 HWT Flag/3(HWT [s])
  HWT_dem [s]/1 -> TIS1 Lead Car Longitudinal Velocity/1(HWT_dem (s)), TIS1 HWT Flag/2(HWT_dem [s])
  TIS1 Objects On Lane/1(TIS1_RANGEDOT [m/s]) -> TIS1 Closest Object/1(TIS1_rangedot [m/s])
  Standstill [m]/1 -> TIS1 Lead Car Longitudinal Velocity/4(Standstill [m]), TIS1 HWT Flag/4(Standstill distance)
  EGO_velocity [m/s]/1 -> TIS1 Lead Car Longitudinal Velocity/3(EGO Velocity [m/s]), TIS1 HWT Computing1/2(Velocity [m/s]), TIS1 HWT Computing/3(Velocity [m/s])
  TIS1 Closest Object/1(rangedot [m/s]) -> TIS1 Lead Car Longitudinal Velocity/2(TIS1 Rangedot [m/s])
  TIS1 Closest Object/2(Distance [m/s]) -> TIS1 Lead distance [m]/1, TIS1 HWT Computing1/1(Distance [m]), TIS1 HWT Flag/1(Distance closest [m])
  HWT_dem [s]1/1 -> TIS1 HWT Computing/2(HWT demanded)
  TIS1 HWT Computing1/1(HWT [s]) -> TIS1_HWT_straight/1
  TIS1 HWT Flag/1(HWT_flag) -> Hold/1(HWTflagIN)
  TIS1 Lead Car Longitudinal Velocity/1(lead_velocity [m/s]) -> Hold/2(lead_vel_in), TIS1 Lead velocity [m/s]/1
  TIS1 Lead Car Longitudinal Velocity/2(Safe distance [m]) -> TIS1 Safe_distance [m]/1
  Hold/1(HWT_flag) -> HWT_flag/1
  TIS1 Objects On Lane/2(TIS1_Distance [m]) -> TIS1 Closest Object/2(TIS1_Distance [m]), TIS1 HWT Computing/1(Distance [m]), TIS1_closest_object_search/1(distance)

== system ACC_speed_change_curve_cs/Audi_A8_1/ACC_System/TIS2 Bend Road ==
  note: === TIS2 Bend Road block ===
      |
      |  - interpretes information provided from the first TIS sensor,
      |  - computes HeadWay Time (HWT) for object on the lane of the EGO car on the bend road,
      |  - determines if detected objects is potentially dengerous,
      |  - outputs distance to the following car, computes its velocity and safe distance to be kept.
  EGO_velocity [m/s] : Inport
  TIS2_range [m] : Inport  Port=2  PortDimensions=TISdet(2)
  TIS2_rangedot [m/s] : Inport  Port=3  PortDimensions=TISdet(2)
  TIS2_theta [deg] : Inport  Port=4  PortDimensions=TISdet(2)
  HWT_dem [s] : Inport  Port=5
  Standstill [m] : Inport  Port=6
  EGO_Yaw_rate [deg/s] : Inport  Port=7
  EGO_velocity [m/s]2 : InportShadow
  Hold : Subsystem
  Lead Car Longitudinal Velocity : Subsystem
  TIS1 HWT Computing : Subsystem
  TIS2 Closest Object On Bend Road : Subsystem
  TIS2 HWT Flag : Subsystem
  TIS2 Objects On Bend Road : Subsystem
  TIS2 Sorting Fun : Subsystem
  TIS2_closest_object_search1 : MATLAB Function  TreatAsAtomicUnit=on
  HWT_flag : Outport
  TIS2 Lead distance [m] : Outport  Port=2
  TIS2 Safe_distance [m] : Outport  Port=3
  TIS2_HWT_bend : Outport  Port=4
  TIS2 Lead velocity [m/s] : Outport  Port=5
  index : Outport  Port=6
  wires:
  TIS2_range [m]/1 -> TIS2 Sorting Fun/1(TIS2range [m])
  TIS2_rangedot [m/s]/1 -> TIS2 Sorting Fun/2(TIS2rangedot [m/s])
  TIS2_theta [deg]/1 -> TIS2 Sorting Fun/3(TIS2theta [deg])
  TIS2 Sorting Fun/1(TIS2_RANGE [m]) -> TIS2 Objects On Bend Road/1(TIS2_range [m])
  TIS2 Sorting Fun/2(TIS2_RANGEDOT [m/s]) -> TIS2 Objects On Bend Road/2(TIS2_rangedot [m/s])
  TIS2 Sorting Fun/3(TIS2_THETA [rad]) -> TIS2 Objects On Bend Road/3(TIS2_theta [rad])
  TIS2 Objects On Bend Road/1(TIS2_RANGE [m]) -> TIS2 Closest Object On Bend Road/2(TIS2_range [m]), TIS2_closest_object_search1/1(distance)
  TIS2 Objects On Bend Road/2(TIS2_RANGEDOT [m/s]) -> TIS2 Closest Object On Bend Road/3(TIS2_rangedot [m])
  TIS2 Objects On Bend Road/3(TIS2_THETA [rad]) -> TIS2 Closest Object On Bend Road/4(TIS2_theta [rad])
  TIS2 Objects On Bend Road/4(TIS1_Distance [m]) -> TIS2 Closest Object On Bend Road/5(TIS2_Distance [m])
  TIS2 Objects On Bend Road/5(TIS2_lambda_[rad]) -> TIS2 Closest Object On Bend Road/6(TIS2_lambda [rad])
  EGO_Yaw_rate [deg/s]/1 -> TIS2 Objects On Bend Road/5(EGO_Yaw_rate_[deg/s])
  EGO_velocity [m/s]/1 -> TIS2 Objects On Bend Road/4(EGO_Velocity [m/s])
  TIS2_closest_object_search1/1(index) -> TIS2 Closest Object On Bend Road/1(index), index/1
  TIS2 Closest Object On Bend Road/3(Distance [m]) -> TIS2 Lead distance [m]/1, TIS2 HWT Flag/1(Distance closest [m]), TIS1 HWT Computing/1(Distance [m])
  EGO_velocity [m/s]2/1 -> TIS1 HWT Computing/2(Velocity [m/s]), Lead Car Longitudinal Velocity/3(EGO Velocity [m/s])
  TIS2 Closest Object On Bend Road/1(rangedot [m/s]) -> Lead Car Longitudinal Velocity/2(TIS1 Rangedot [m/s])
  HWT_dem [s]/1 -> Lead Car Longitudinal Velocity/1(HWT_dem (s)), TIS2 HWT Flag/3(HWT_dem [s])
  TIS1 HWT Computing/1(HWT [s]) -> TIS2_HWT_bend/1, TIS2 HWT Flag/2(HWT [s])
  Standstill [m]/1 -> Lead Car Longitudinal Velocity/4(Standstill [m]), TIS2 HWT Flag/4(Standstill distance)
  TIS2 Closest Object On Bend Road/5(lambda [rad]) -> Lead Car Longitudinal Velocity/6(lambda [rad])
  TIS2 Closest Object On Bend Road/2(theta [rad]) -> Lead Car Longitudinal Velocity/5(theta [rad])
  TIS2 Closest Object On Bend Road/4(range [m]) -> Lead Car Longitudinal Velocity/7(TIS2 Range [m])
  Lead Car Longitudinal Velocity/1(Safe distance [m]) -> TIS2 Safe_distance [m]/1
  Lead Car Longitudinal Velocity/2(Lead velocity [m/s]) -> TIS2 Lead velocity [m/s]/1, Hold/2(lead_vel_in)
  Hold/1(HWT_flag) -> HWT_flag/1
  TIS2 HWT Flag/1(HWT_flag) -> Hold/1(HWTflagIN)
